simulink model "three_level_h_brige_inverter"  (R2021a)
settings: Solver=ode4  StartTime=0.0  StopTime=0.1  FixedStep=1e-6  RelTol=1e-3
libraries: spsIGBTDiodeLib x4, simulink x2, spsDCVoltageSourceLib x1, spsVoltageMeasurementLib x1, spspowerguiLib x1
settings Model: Creator=PRANAY KAMAL  LastModifiedBy=PRANAY KAMAL
settings DataIOCC: ReturnWorkspaceOutputs=off

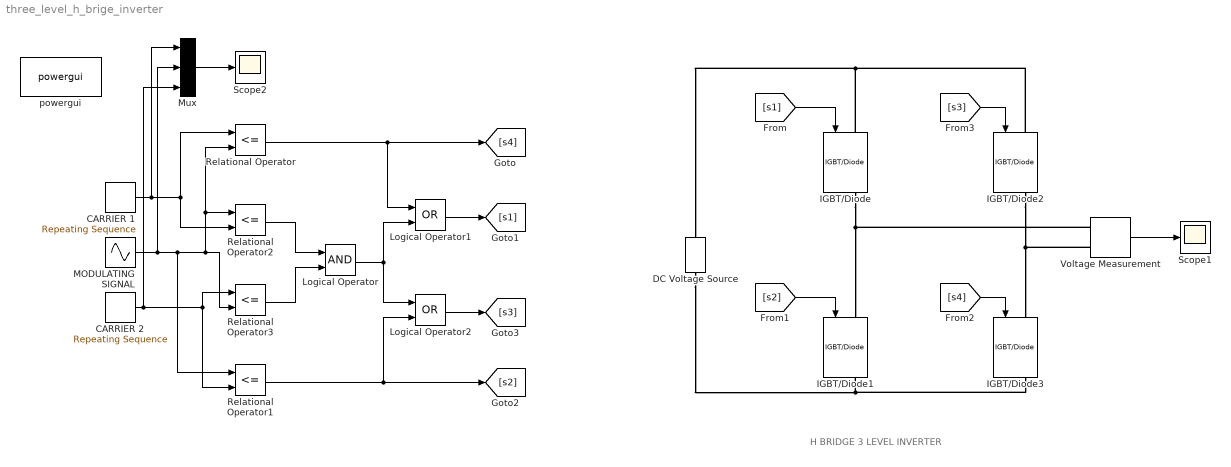
== system three_level_h_brige_inverter ==
  note: H BRIDGE 3 LEVEL INVERTER
  CARRIER 1 : simulink/Sources/Repeating Sequence  rep_seq_t=[0 0.5 1]*(1/6000)  rep_seq_y=[0 1 0]
  CARRIER 2 : simulink/Sources/Repeating Sequence  rep_seq_t=[0 0.5 1]*(1/6000)  rep_seq_y=[-1 0 -1]
  DC Voltage Source : spsDCVoltageSourceLib/DC Voltage Source  Amplitude=400  Measurements=None
  IGBT/Diode{,1..3} (4 alike) : spsIGBTDiodeLib/IGBT//Diode  Ron=1e-3  Rs=1e5  Cs=inf  Measurements=on
  Logical Operator : Logic  AllPortsSameDT=off  OutDataTypeStr=boolean
  Logical Operator1 : Logic  Operator=OR  AllPortsSameDT=off  OutDataTypeStr=boolean
  Logical Operator2 : Logic  Operator=OR  AllPortsSameDT=off  OutDataTypeStr=boolean
  MODULATING SIGNAL : Sin  Amplitude=0.8  Frequency=2*pi*60  SampleTime=0
  Mux : Mux  Inputs=3
  Relational Operator{,1..3} (4 alike) : RelationalOperator  Operator=<=  OutDataTypeStr=boolean  RndMeth=Simplest
  Scope1 : Scope
  Scope2 : Scope
  Voltage Measurement : spsVoltageMeasurementLib/Voltage Measurement  PhasorSimulation=off  OutputType=Complex  PSBequivalent=0
  powergui : spspowerguiLib/powergui  Priority=1  SimulationMode=Continuous  SampleTime=50e-6  frequency=60  Iterations=50  frequencyindice=0  Pbase=100e6  ErrMax=1e-4  UnitsV=kV  UnitsW=MW  buscounter=0  FunctionMessages=off  echomessages=off  EnableUseOfTLC=off  CurrentSourceSwitches=off  DisableSnubberDevices=off  DisableRonSwitches=off  DisableVfSwitches=off  DisplayEquations=off  AutomaticDiscreteSolvers=off  SolverType=Tustin/Backward Euler (TBE)  Interpol=off  ExternalGateDelay=off  methode=off  Ts=100  x0status=blocks  SPID=on  SwTol=0  HookPort=off  NonlinearTolerance=1e-4  nMaxIteration=100  ContinueOnMaxIteration=off  RestoreLinks=warning  ResistiveCurrentMeasurement=off  Frange=[0:2:500]  Ylog=off  Xlog=on  ShowGrid=off  save=off  variable=ZData  structure=0  ZoomFFT=off  StartTime=0.0  cycles=1  DisplayStyle=1  fundamental=60  FreqAxis=off  MaxFrequency=1000  frequencyindicesteady=1  RmsSteady=1  display=off
  wires:
  CARRIER 1/1 -> Mux/1, Relational Operator2/2, Relational Operator/1
  MODULATING SIGNAL/1 -> Mux/2, Relational Operator3/2, Relational Operator2/1, Relational Operator/2, Relational Operator1/1
  CARRIER 2/1 -> Relational Operator1/2, Relational Operator3/1, Mux/3
  Relational Operator2/1 -> Logical Operator/1
  Relational Operator3/1 -> Logical Operator/2
  Relational Operator1/1 -> Logical Operator2/2, [s2]
  Relational Operator/1 -> Logical Operator1/1, [s4]
  Mux/1 -> Scope2/1
  [s1] -> IGBT/Diode/1
  [s2] -> IGBT/Diode1/1
  [s4] -> IGBT/Diode3/1
  [s3] -> IGBT/Diode2/1
  Logical Operator/1 -> Logical Operator2/1, Logical Operator1/2
  Logical Operator1/1 -> [s1]
  Logical Operator2/1 -> [s3]
  Voltage Measurement/1 -> Scope1/1
  connections:
  IGBT/Diode/RConn1 -- Voltage Measurement/LConn1 -- IGBT/Diode1/LConn1
  IGBT/Diode2/RConn1 -- Voltage Measurement/LConn2 -- IGBT/Diode3/LConn1
  IGBT/Diode/LConn1 -- DC Voltage Source/RConn1 -- IGBT/Diode2/LConn1
  DC Voltage Source/LConn1 -- IGBT/Diode3/RConn1 -- IGBT/Diode1/RConn1
